simulink model "planLocal_simfcn"  (R2024b)
settings: Solver=FixedStepDiscrete  StartTime=0.0  StopTime=30  RelTol=1e-3
InitFcn:
  | localPlanSetup
undefined symbols (not defined in the file): n, refPath, tuneableTEBParamsCpp, worldGridLoc, worldMat, worldRes
libraries: roshelperlib x2, simulink x1
settings Model: Creator=cstabile  LastModifiedBy=jbrault
settings SolverCC: DateTimeAtSimulationTimeZero=[]
settings SFSimCC: SimTargetLang=C++

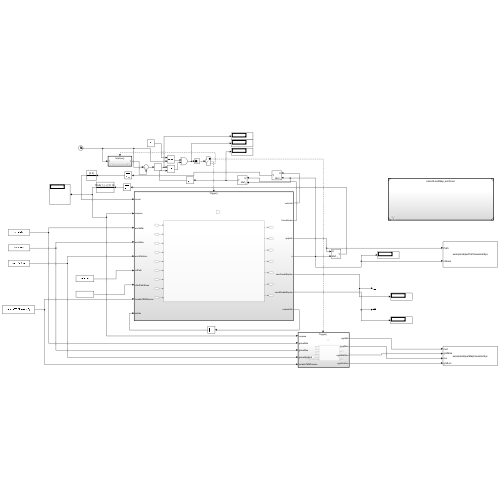
[thumbnail: Simulink's stored preview of the top-level diagram]
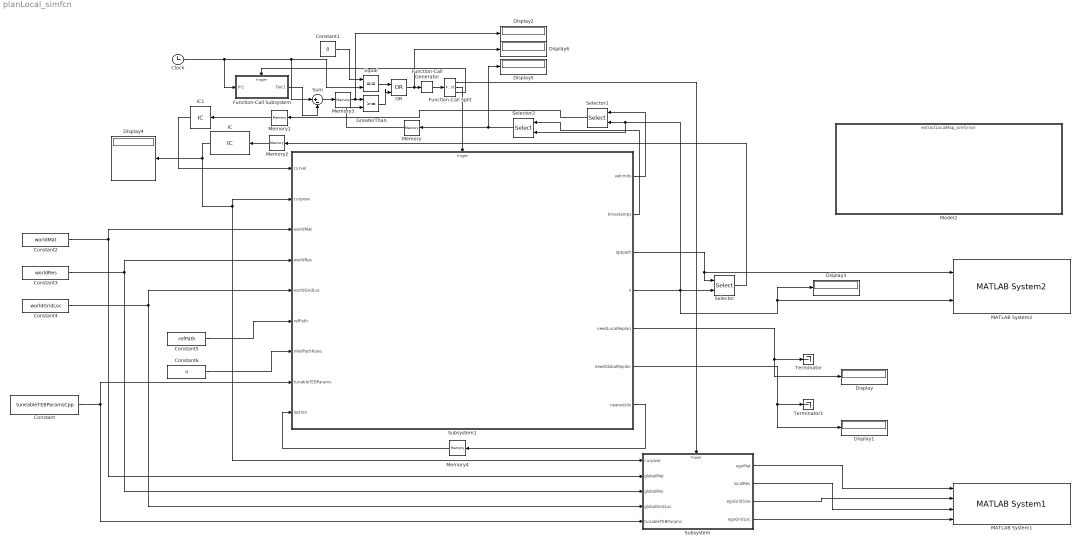
== system planLocal_simfcn ==
  Clock : Clock
  Constant : Constant  Value=tuneableTEBParamsCpp  OutDataTypeStr=Bus: teb_bus
  Constant1 : Constant  Value=0
  Constant2 : Constant  Value=worldMat  VectorParams1D=off
  Constant3 : Constant  Value=worldRes
  Constant4 : Constant  Value=worldGridLoc  VectorParams1D=off
  Constant5 : Constant  Value=refPath  VectorParams1D=off
  Constant6 : Constant  Value=n
  Display{,1..6} (7 alike) : Display
  Equal : RelationalOperator  Operator===  OutDataTypeStr=boolean  RndMeth=Simplest  InputSameDT=off
  Function-Call Generator : simulink/Ports & Subsystems/Function-Call Generator  sample_time=1  numberOfIterations=1  DisallowWideOutput=off  ShowEnablePort=on
  Function-Call Split : FunctionCallSplit  IconShape=distinctive  NumOutputPorts=3  OutputPortLayout=default
  Function-Call Subsystem : Subsystem  TreatAsAtomicUnit=on
  GreaterThan : RelationalOperator  OutDataTypeStr=boolean  RndMeth=Simplest  InputSameDT=off
  IC : InitialCondition  Value=refPath(1,:) + [10 10 0]
  IC1 : InitialCondition  Value=[0 0]
  MATLAB System1 : roshelperlib/MATLAB System1  MapType=SDF  IsEgo=off  DisplayVisual=on  SimulateUsing=Interpreted execution
  MATLAB System2 : roshelperlib/MATLAB System2  VisualizationParameters={'k-'}  PlotType=Line  DisplayVisual=on  SimulateUsing=Interpreted execution
  Memory{,1..4} (5 alike) : Memory
  Model2 : ModelReference  ModelNameDialog=extractLocalMap_simfcnsvr.slx  SimulationMode=Normal  ScheduleRates=on  ModelReferenceVersion=2.0
  OR : Logic  Operator=OR  IconShape=distinctive  AllPortsSameDT=off  OutDataTypeStr=boolean
  Selector : Selector  NumberOfDimensions=2  InputPortWidth=3  IndexOptions=Starting index (port),Select all  Indices=[1 3],1  OutputSizes=1,1
  Selector1 : Selector  NumberOfDimensions=2  InputPortWidth=3  IndexOptions=Starting index (port),Select all  Indices=[1 3],1  OutputSizes=1,1
  Selector2 : Selector  NumberOfDimensions=2  InputPortWidth=3  IndexOptions=Starting index (port),Select all  Indices=[1 3],1  OutputSizes=1,1
  Subsystem : Subsystem
  Subsystem1 : Subsystem
  Sum : Sum  Inputs=|+-
  Terminator : Terminator
  Terminator1 : Terminator
  wires:
  Clock/1 -> Function-Call Subsystem/1(In1), Sum/1, Equal/2
  GreaterThan/1 -> OR/2
  Equal/1 -> OR/1
  Constant1/1 -> Equal/1
  OR/1 -> Display6/1, Function-Call Generator/1
  Selector/1 -> Memory2/1
  Constant2/1 -> Subsystem1/3(worldMat), Subsystem/2(globalMat)
  Constant3/1 -> Subsystem1/4(worldRes), Subsystem/3(globalRes)
  Constant4/1 -> Subsystem1/5(worldGridLoc), Subsystem/4(globalGridLoc)
  Constant/1 -> Subsystem/5(tunableTEBParams), Subsystem1/8(tunableTEBParams)
  Function-Call Split/2 -> Subsystem1/Trigger
  IC/1 -> Subsystem1/2(curpose), Subsystem/1(curpose), Display4/1
  Selector1/1 -> Memory1/1
  Function-Call Generator/1 -> Function-Call Split/1
  Selector2/1 -> Display5/1, Memory/1
  Function-Call Split/1 -> Subsystem/Trigger
  Memory/1 -> GreaterThan/2
  Memory1/1 -> IC1/1
  Memory2/1 -> IC/1
  Function-Call Split/3 -> Function-Call Subsystem/Trigger
  Function-Call Subsystem/1(Out1) -> Sum/2
  Sum/1 -> Memory3/1
  Memory3/1 -> Display2/1, GreaterThan/1
  Subsystem/1(egoMat) -> MATLAB System1/1
  Subsystem/2(localRes) -> MATLAB System1/3
  Subsystem/3(egoGridSize) -> MATLAB System1/2
  Subsystem/4(egoGridLoc) -> MATLAB System1/4
  Subsystem1/5(needLocalReplan) -> Display/1, Terminator/1
  Subsystem1/3(optpath) -> Selector/1, MATLAB System2/1
  Subsystem1/6(needGlobalReplan) -> Display1/1, Terminator1/1
  Subsystem1/4(n) -> Display3/1, MATLAB System2/2, Selector/2, Selector2/2, Selector1/2
  IC1/1 -> Subsystem1/1(curvel)
  Constant5/1 -> Subsystem1/6(refPath)
  Constant6/1 -> Subsystem1/7(nRefPathRows)
  Subsystem1/1(velcmds) -> Selector1/1
  Subsystem1/2(timestamps) -> Selector2/1
  Subsystem1/7(nearestIdx) -> Memory4/1
  Memory4/1 -> Subsystem1/9(lastIdx)

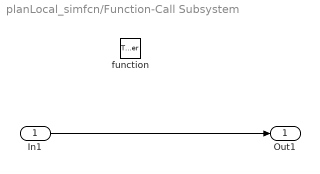
== system planLocal_simfcn/Function-Call Subsystem ==
  In1 : Inport
  function : TriggerPort  TriggerType=function-call  VariantControl=(inherit)
  Out1 : Outport
  wires:
  In1/1 -> Out1/1

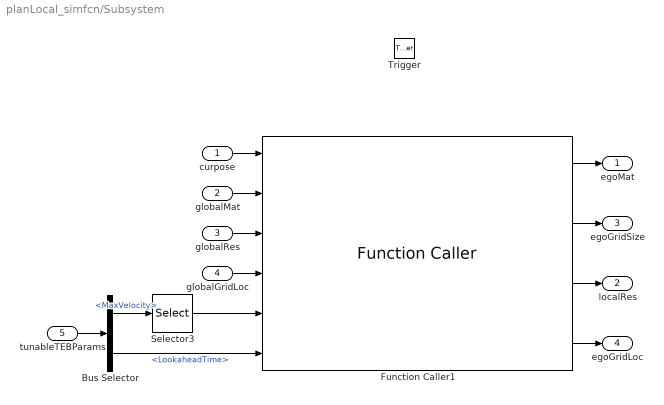
== system planLocal_simfcn/Subsystem ==
  curpose : Inport
  globalMat : Inport  Port=2
  globalRes : Inport  Port=3
  globalGridLoc : Inport  Port=4
  tunableTEBParams : Inport  Port=5
  Trigger : TriggerPort  TriggerType=function-call  VariantControl=(inherit)  PortDimensions=1
  Bus Selector : BusSelector  OutputSignals=MaxVelocity,LookaheadTime
  Function Caller1 : FunctionCaller  FunctionPrototype=[egoMat,egoGridSize,localRes,egoGridLoc] = extractLocalMap(curpose,globalMat,globalRes,globalGridLoc,maxVel,lookaheadTime)  InputArgumentSpecifications=<Enter example>  OutputArgumentSpecifications=<Enter example>
  Selector3 : Selector  InputPortWidth=2  IndexOptions=Index vector (dialog)  Indices=1  OutputSizes=1
  egoMat : Outport
  localRes : Outport  Port=2
  egoGridSize : Outport  Port=3
  egoGridLoc : Outport  Port=4
  wires:
  Selector3/1 -> Function Caller1/5
  tunableTEBParams/1 -> Bus Selector/1
  globalGridLoc/1 -> Function Caller1/4
  globalMat/1 -> Function Caller1/2
  Bus Selector/1 -> Selector3/1  "<MaxVelocity>"
  Bus Selector/2 -> Function Caller1/6  "<LookaheadTime>"
  curpose/1 -> Function Caller1/1
  globalRes/1 -> Function Caller1/3
  Function Caller1/1 -> egoMat/1
  Function Caller1/2 -> egoGridSize/1
  Function Caller1/3 -> localRes/1
  Function Caller1/4 -> egoGridLoc/1

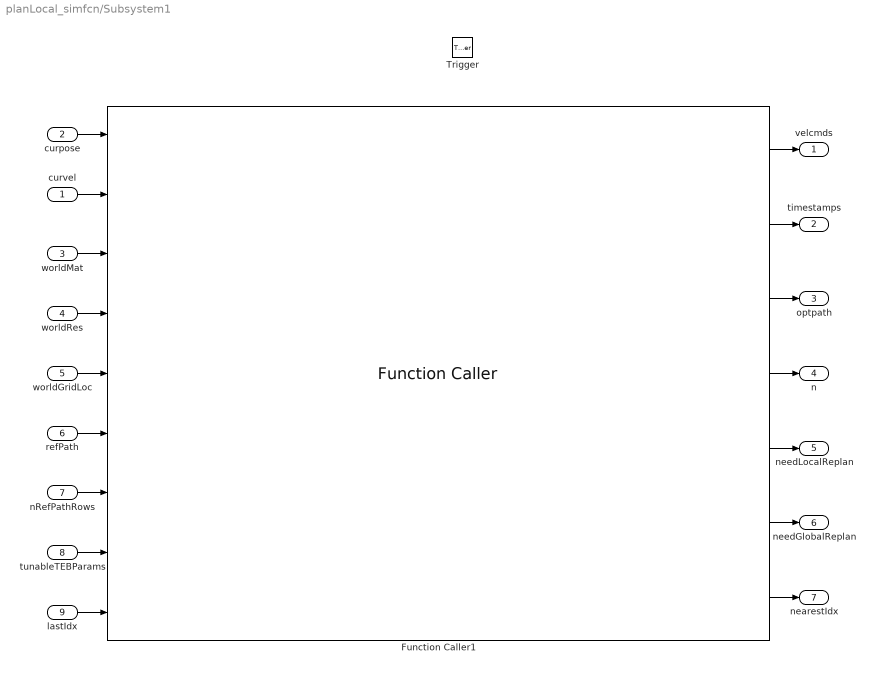
== system planLocal_simfcn/Subsystem1 ==
  curvel : Inport
  curpose : Inport  Port=2
  worldMat : Inport  Port=3
  worldRes : Inport  Port=4
  worldGridLoc : Inport  Port=5
  refPath : Inport  Port=6
  nRefPathRows : Inport  Port=7
  tunableTEBParams : Inport  Port=8
  lastIdx : Inport  Port=9
  Trigger : TriggerPort  TriggerType=function-call  VariantControl=(inherit)  PortDimensions=1
  Function Caller1 : FunctionCaller  FunctionPrototype=[velcmds,timestamps,optpath,n,needLocalReplan,needGlobalReplan,nearestIdx] = planLocal(curpose,curvel,worldMat,worldRes,worldGridLoc,refPathXY,nRefPathrows,tuneableTEBParams,lastIdx)  InputArgumentSpecifications=<Enter example>  OutputArgumentSpecifications=<Enter example>
  velcmds : Outport
  timestamps : Outport  Port=2
  optpath : Outport  Port=3
  n : Outport  Port=4
  needLocalReplan : Outport  Port=5
  needGlobalReplan : Outport  Port=6
  nearestIdx : Outport  Port=7
  wires:
  worldRes/1 -> Function Caller1/4
  curpose/1 -> Function Caller1/1
  worldMat/1 -> Function Caller1/3
  curvel/1 -> Function Caller1/2
  nRefPathRows/1 -> Function Caller1/7
  worldGridLoc/1 -> Function Caller1/5
  tunableTEBParams/1 -> Function Caller1/8
  refPath/1 -> Function Caller1/6
  Function Caller1/1 -> velcmds/1
  Function Caller1/2 -> timestamps/1
  Function Caller1/3 -> optpath/1
  Function Caller1/4 -> n/1
  Function Caller1/5 -> needLocalReplan/1
  Function Caller1/6 -> needGlobalReplan/1
  lastIdx/1 -> Function Caller1/9
  Function Caller1/7 -> nearestIdx/1
